simulink model "motor_model"  (R2017a)
settings: Solver=ode45  StartTime=0.0  StopTime=20  RelTol=1e-3  EnableMultiTasking=on
values from neighbouring files (symbols this model uses):
  motor = gm9434    [motor_code.m]
undefined symbols (not defined in the file or in its folder): current_ctrl, joint, position_ctrl, speed_ctrl, vest
libraries: simulink x3
settings Model: Creator=rodrigo  LastModifiedBy=rodrigo
settings DataIOCC: LimitDataPoints=on  SaveFormat=Array
settings OptimizationCC: LifeSpan=inf
settings DebuggingCC: UnderspecifiedInitializationDetection=Classic  MergeDetectMultiDrivingBlocksExec=none  StateNameClashWarn=warning  SFUnexpectedBacktrackingDiag=warning  SFNoUnconditionalDefaultTransitionDiag=warning  SFExecutionAtInitializationDiag=none
settings HardwareCC: ProdBitPerPointer=32  ProdBitPerSizeT=32  ProdBitPerPtrDiffT=32  ProdLargestAtomicFloat=None  ProdIntDivRoundTo=Undefined  ProdEndianess=Unspecified  ProdWordSize=32  ProdHWDeviceType=32-bit Generic
settings ModelReferenceCC: PropagateSignalLabelsOutOfModel=off
settings GRTTargetCC: TargetLangStandard=C89/C90 (ANSI)  GeneratePreprocessorConditionals=Disable all
settings ConfigComp: CovMetricSettings=dw  CovHtmlReporting=on  CovSaveCumulativeToWorkspaceVar=on  CovSaveSingleToWorkspaceVar=on  CovExternalEMLEnable=off

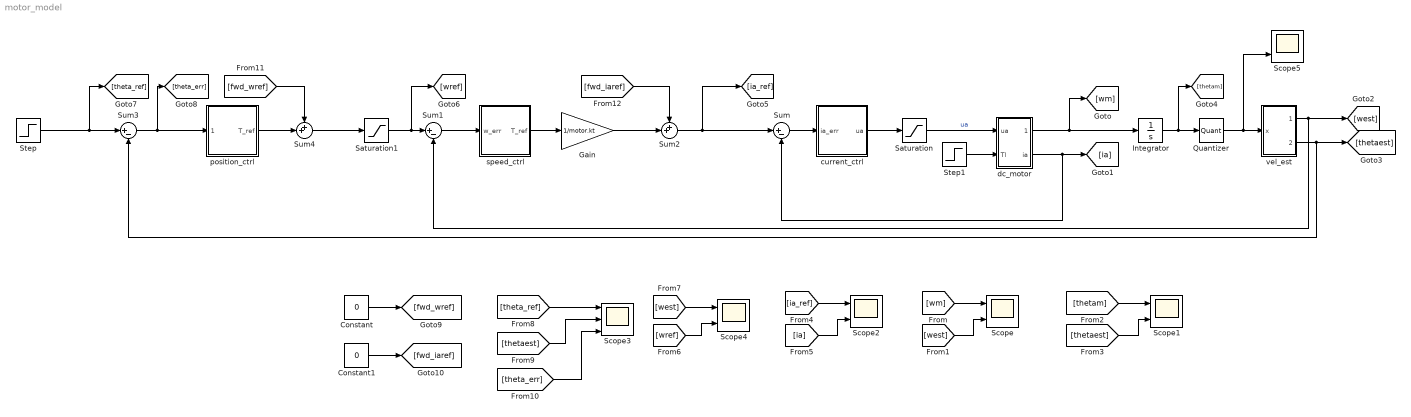
== system motor_model ==
  Constant : Constant  Value=0
  Constant1 : Constant  Value=0
  Gain : Gain  Gain=1/motor.kt
  Integrator : Integrator
  Quantizer : Quantizer  QuantizationInterval=encoder
  Saturation : Saturate  UpperLimit=12  LowerLimit=-12
  Saturation1 : Saturate  UpperLimit=motor.max_speed  LowerLimit=-motor.max_speed
  Scope{,1..2,4..5} (5 alike) : Scope  NumInputPorts=2
  Scope3 : Scope  NumInputPorts=3
  Step : Step  After=800  SampleTime=0
  Step1 : Step  After=0  SampleTime=0  ZeroCross=off
  Sum : Sum  Inputs=|+-
  Sum1 : Sum  Inputs=|+-
  Sum2 : Sum  Inputs=++|
  Sum3 : Sum  Inputs=|+-
  Sum4 : Sum  Inputs=++|
  current_ctrl : Subsystem
  dc_motor : Subsystem
  position_ctrl : Subsystem
  speed_ctrl : Subsystem
  vel_est : Subsystem
  wires:
  [wm] -> Scope/1
  [west] -> Scope/2
  dc_motor/2(ia) -> [ia], Sum/2
  Step1/1 -> dc_motor/2(Tl)
  Saturation/1 -> dc_motor/1(ua)  "ua"
  dc_motor/1(wm) -> Integrator/1, [wm]
  Integrator/1 -> Quantizer/1, [thetam]
  Quantizer/1 -> Scope5/2, vel_est/1(x)
  [thetam] -> Scope1/1
  [thetaest] -> Scope1/2
  vel_est/2(xest) -> Sum3/2, [thetaest]
  [ia_ref] -> Scope2/1
  [ia] -> Scope2/2
  Sum/1 -> current_ctrl/1(ia_err)
  current_ctrl/1(ua) -> Saturation/1
  speed_ctrl/1(T_ref) -> Gain/1
  Sum1/1 -> speed_ctrl/1(w_err)
  [west] -> Scope4/1
  [wref] -> Scope4/2
  Sum2/1 -> [ia_ref], Sum/1
  Gain/1 -> Sum2/2
  [fwd_iaref] -> Sum2/1
  Step/1 -> [theta_ref], Sum3/1
  Sum3/1 -> [theta_err], position_ctrl/1(theta_err)
  [theta_ref] -> Scope3/1
  [theta_err] -> Scope3/3
  vel_est/1(vest) -> Sum1/2, [west]
  [thetaest] -> Scope3/2
  Saturation1/1 -> [wref], Sum1/1
  [fwd_wref] -> Sum4/1
  position_ctrl/1(T_ref) -> Sum4/2
  Sum4/1 -> Saturation1/1
  Constant/1 -> [fwd_wref]
  Constant1/1 -> [fwd_iaref]

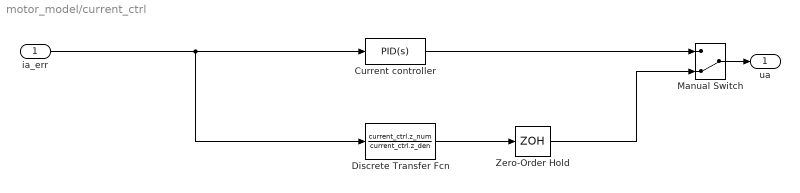
== system motor_model/current_ctrl ==
  ia_err : Inport
  Current controller : simulink/Continuous/PID Controller  Controller=PID  TimeDomain=Continuous-time  SampleTime=-1  IntegratorMethod=Forward Euler  FilterMethod=Forward Euler  Form=Parallel  UseFilter=off  ControllerParametersSource=internal  P=current_ctrl.kp  I=current_ctrl.ki  D=0  N=100  InitialConditionSource=internal  InitialConditionForIntegrator=0  InitialConditionForFilter=0  ExternalReset=none  ZeroCross=off  LimitOutput=on  UpperSaturationLimit=12  LowerSaturationLimit=-12  LinearizeAsGain=off  AntiWindupMode=back-calculation  Kb=1  TrackingMode=off  Kt=1  PParamMin=[]  PParamMax=[]  IParamMin=[]  IParamMax=[]  DParamMin=[]  DParamMax=[]  NParamMin=[]  NParamMax=[]  KbParamMin=[]  KbParamMax=[]  KtParamMin=[]  KtParamMax=[]  POutMin=[]  POutMax=[]  IOutMin=[]  IOutMax=[]  DOutMin=[]  DOutMax=[]  NOutMin=[]  NOutMax=[]  KbOutMin=[]  KbOutMax=[]  KtOutMin=[]  KtOutMax=[]  IntegratorOutMin=[]  IntegratorOutMax=[]  FilterOutMin=[]  FilterOutMax=[]  SumOutMin=[]  SumOutMax=[]  SumI1OutMin=[]  SumI1OutMax=[]  SumI2OutMin=[]  SumI2OutMax=[]  SumI3OutMin=[]  SumI3OutMax=[]  SumDOutMin=[]  SumDOutMax=[]  SaturationOutMin=[]  SaturationOutMax=[]  IntegratorContinuousStateAttributes=''  IntegratorStateMustResolveToSignalObject=off  IntegratorRTWStateStorageClass=Auto  FilterContinuousStateAttributes=''  FilterStateMustResolveToSignalObject=off  FilterRTWStateStorageClass=Auto  DifferentiatorICPrevScaledInput=0  DifferentiatorOutMin=[]  DifferentiatorOutMax=[]  InitialConditionSetting=State (most efficient)
  Discrete Transfer Fcn : DiscreteTransferFcn  Numerator=current_ctrl.z_num  Denominator=current_ctrl.z_den  SampleTime=current_ctrl.Ts
  Manual Switch : ManualSwitch  CurrentSetting=0
  Zero-Order Hold : ZeroOrderHold  SampleTime=-1
  ua : Outport
  wires:
  ia_err/1 -> Discrete Transfer Fcn/1, Current controller/1
  Current controller/1 -> Manual Switch/1
  Discrete Transfer Fcn/1 -> Zero-Order Hold/1
  Zero-Order Hold/1 -> Manual Switch/2
  Manual Switch/1 -> ua/1

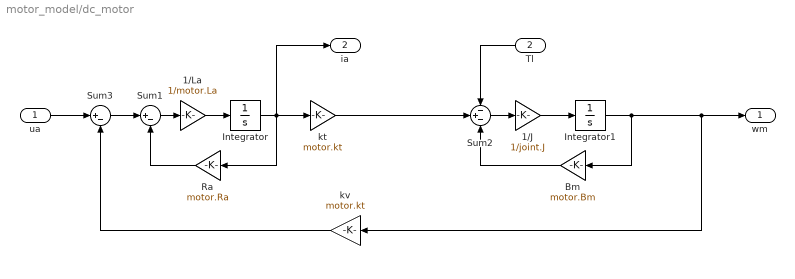
== system motor_model/dc_motor ==
  ua : Inport
  Tl : Inport  Port=2
  1/J : Gain  Gain=1/joint.J
  1/La : Gain  Gain=1/motor.La
  Bm : Gain  Gain=motor.Bm
  Integrator : Integrator  ZeroCross=off
  Integrator1 : Integrator
  Ra : Gain  Gain=motor.Ra
  Sum1 : Sum  Inputs=|+-
  Sum2 : Sum  Inputs=-+-
  Sum3 : Sum  Inputs=|+-
  kt : Gain  Gain=motor.kt
  kv : Gain  Gain=motor.kt
  wm : Outport
  ia : Outport  Port=2
  wires:
  1/J/1 -> Integrator1/1
  Sum2/1 -> 1/J/1
  Integrator1/1 -> Bm/1, wm/1, kv/1
  ua/1 -> Sum3/1
  Integrator/1 -> kt/1, Ra/1, ia/1
  Ra/1 -> Sum1/2
  1/La/1 -> Integrator/1
  Tl/1 -> Sum2/1
  kv/1 -> Sum3/2
  Sum3/1 -> Sum1/1
  Sum1/1 -> 1/La/1
  kt/1 -> Sum2/2
  Bm/1 -> Sum2/3

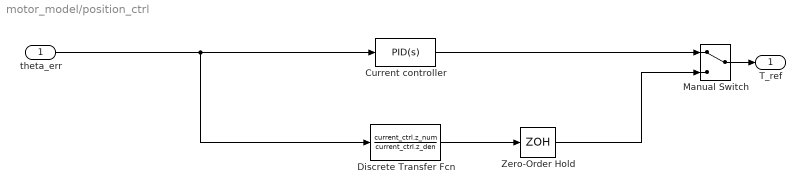
== system motor_model/position_ctrl ==
  theta_err : Inport
  Current controller : simulink/Continuous/PID Controller  Controller=PID  TimeDomain=Continuous-time  SampleTime=-1  IntegratorMethod=Forward Euler  FilterMethod=Forward Euler  Form=Ideal  UseFilter=off  ControllerParametersSource=internal  P=position_ctrl.kp  I=0  D=0  N=100  InitialConditionSource=internal  InitialConditionForIntegrator=0  InitialConditionForFilter=0  ExternalReset=none  ZeroCross=off  LimitOutput=off  UpperSaturationLimit=300  LowerSaturationLimit=-300  LinearizeAsGain=off  AntiWindupMode=clamping  Kb=1  TrackingMode=off  Kt=1  PParamMin=[]  PParamMax=[]  IParamMin=[]  IParamMax=[]  DParamMin=[]  DParamMax=[]  NParamMin=[]  NParamMax=[]  KbParamMin=[]  KbParamMax=[]  KtParamMin=[]  KtParamMax=[]  POutMin=[]  POutMax=[]  IOutMin=[]  IOutMax=[]  DOutMin=[]  DOutMax=[]  NOutMin=[]  NOutMax=[]  KbOutMin=[]  KbOutMax=[]  KtOutMin=[]  KtOutMax=[]  IntegratorOutMin=[]  IntegratorOutMax=[]  FilterOutMin=[]  FilterOutMax=[]  SumOutMin=[]  SumOutMax=[]  SumI1OutMin=[]  SumI1OutMax=[]  SumI2OutMin=[]  SumI2OutMax=[]  SumI3OutMin=[]  SumI3OutMax=[]  SumDOutMin=[]  SumDOutMax=[]  SaturationOutMin=[]  SaturationOutMax=[]  IntegratorContinuousStateAttributes=''  IntegratorStateMustResolveToSignalObject=off  IntegratorRTWStateStorageClass=Auto  FilterContinuousStateAttributes=''  FilterStateMustResolveToSignalObject=off  FilterRTWStateStorageClass=Auto  DifferentiatorICPrevScaledInput=0  DifferentiatorOutMin=[]  DifferentiatorOutMax=[]  InitialConditionSetting=State (most efficient)
  Discrete Transfer Fcn : DiscreteTransferFcn  Numerator=current_ctrl.z_num  Denominator=current_ctrl.z_den  SampleTime=current_ctrl.Ts
  Manual Switch : ManualSwitch
  Zero-Order Hold : ZeroOrderHold  SampleTime=-1
  T_ref : Outport
  wires:
  theta_err/1 -> Current controller/1, Discrete Transfer Fcn/1
  Current controller/1 -> Manual Switch/1
  Discrete Transfer Fcn/1 -> Zero-Order Hold/1
  Zero-Order Hold/1 -> Manual Switch/2
  Manual Switch/1 -> T_ref/1

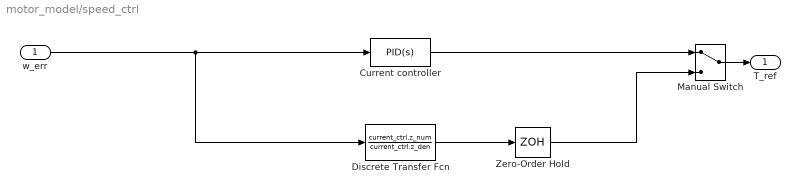
== system motor_model/speed_ctrl ==
  w_err : Inport
  Current controller : simulink/Continuous/PID Controller  Controller=PID  TimeDomain=Continuous-time  SampleTime=-1  IntegratorMethod=Forward Euler  FilterMethod=Forward Euler  Form=Ideal  UseFilter=off  ControllerParametersSource=internal  P=speed_ctrl.kp  I=speed_ctrl.ki  D=0  N=100  InitialConditionSource=internal  InitialConditionForIntegrator=0  InitialConditionForFilter=0  ExternalReset=none  ZeroCross=off  LimitOutput=on  UpperSaturationLimit=3  LowerSaturationLimit=-3  LinearizeAsGain=off  AntiWindupMode=back-calculation  Kb=1  TrackingMode=off  Kt=1  PParamMin=[]  PParamMax=[]  IParamMin=[]  IParamMax=[]  DParamMin=[]  DParamMax=[]  NParamMin=[]  NParamMax=[]  KbParamMin=[]  KbParamMax=[]  KtParamMin=[]  KtParamMax=[]  POutMin=[]  POutMax=[]  IOutMin=[]  IOutMax=[]  DOutMin=[]  DOutMax=[]  NOutMin=[]  NOutMax=[]  KbOutMin=[]  KbOutMax=[]  KtOutMin=[]  KtOutMax=[]  IntegratorOutMin=[]  IntegratorOutMax=[]  FilterOutMin=[]  FilterOutMax=[]  SumOutMin=[]  SumOutMax=[]  SumI1OutMin=[]  SumI1OutMax=[]  SumI2OutMin=[]  SumI2OutMax=[]  SumI3OutMin=[]  SumI3OutMax=[]  SumDOutMin=[]  SumDOutMax=[]  SaturationOutMin=[]  SaturationOutMax=[]  IntegratorContinuousStateAttributes=''  IntegratorStateMustResolveToSignalObject=off  IntegratorRTWStateStorageClass=Auto  FilterContinuousStateAttributes=''  FilterStateMustResolveToSignalObject=off  FilterRTWStateStorageClass=Auto  DifferentiatorICPrevScaledInput=0  DifferentiatorOutMin=[]  DifferentiatorOutMax=[]  InitialConditionSetting=State (most efficient)
  Discrete Transfer Fcn : DiscreteTransferFcn  Numerator=current_ctrl.z_num  Denominator=current_ctrl.z_den  SampleTime=current_ctrl.Ts
  Manual Switch : ManualSwitch
  Zero-Order Hold : ZeroOrderHold  SampleTime=-1
  T_ref : Outport
  wires:
  w_err/1 -> Current controller/1, Discrete Transfer Fcn/1
  Current controller/1 -> Manual Switch/1
  Discrete Transfer Fcn/1 -> Zero-Order Hold/1
  Zero-Order Hold/1 -> Manual Switch/2
  Manual Switch/1 -> T_ref/1

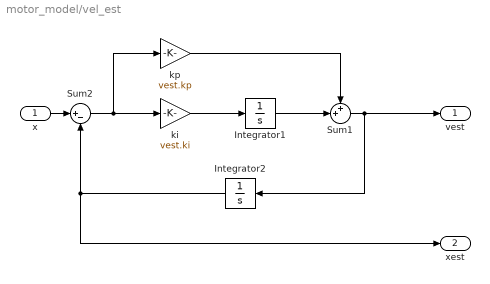
== system motor_model/vel_est ==
  x : Inport
  Integrator1 : Integrator
  Integrator2 : Integrator
  Sum1 : Sum  Inputs=++|
  Sum2 : Sum  Inputs=|+-
  ki : Gain  Gain=vest.ki
  kp : Gain  Gain=vest.kp
  vest : Outport
  xest : Outport  Port=2
  wires:
  ki/1 -> Integrator1/1
  Sum2/1 -> kp/1, ki/1
  Integrator2/1 -> xest/1, Sum2/2
  kp/1 -> Sum1/1
  Integrator1/1 -> Sum1/2
  x/1 -> Sum2/1
  Sum1/1 -> vest/1, Integrator2/1
